simulink model "Kontrol"  (R2022a)
settings: Solver=FixedStepAuto  StartTime=0.0  StopTime=1.0  FixedStep=1/25e3  RelTol=1e-3
settings Model: Creator=unaly  LastModifiedBy=unaly

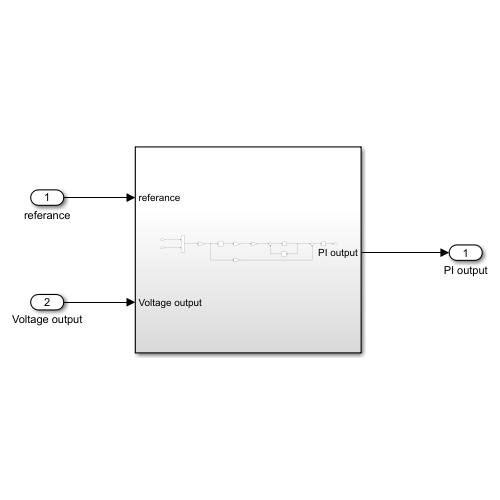
[thumbnail: Simulink's stored preview of the top-level diagram]
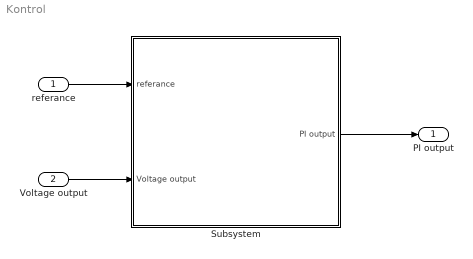
== system Kontrol ==
  referance : Inport
  Voltage output : Inport  Port=2
  Subsystem : Subsystem
  PI output : Outport
  wires:
  referance/1 -> Subsystem/1(referance)
  Voltage output/1 -> Subsystem/2(Voltage output)
  Subsystem/1(PI output) -> PI output/1

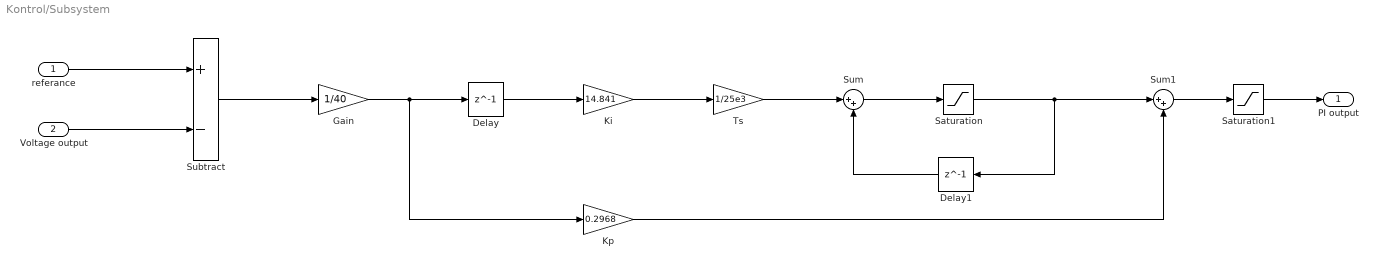
== system Kontrol/Subsystem ==
  referance : Inport
  Voltage output : Inport  Port=2
  Delay : Delay  DelayLength=1
  Delay1 : Delay  DelayLength=1
  Gain : Gain  Gain=1/40
  Ki : Gain  Gain=14.841
  Kp : Gain  Gain=0.2968
  Saturation : Saturate  UpperLimit=0.99  LowerLimit=0.01
  Saturation1 : Saturate  UpperLimit=0.99  LowerLimit=0.01
  Subtract : Sum  Inputs=+-
  Sum : Sum  Inputs=|++
  Sum1 : Sum  Inputs=|++
  Ts : Gain  Gain=1/25e3
  PI output : Outport
  wires:
  Sum1/1 -> Saturation1/1
  Sum/1 -> Saturation/1
  Saturation/1 -> Delay1/1, Sum1/1
  Delay/1 -> Ki/1
  referance/1 -> Subtract/1
  Voltage output/1 -> Subtract/2
  Gain/1 -> Kp/1, Delay/1
  Subtract/1 -> Gain/1
  Ts/1 -> Sum/1
  Ki/1 -> Ts/1
  Kp/1 -> Sum1/2
  Delay1/1 -> Sum/2
  Saturation1/1 -> PI output/1
